simulink model "multipercursorealey"  (R2015a)
settings: Solver=ode45  StartTime=0.0  StopTime=1000.0  RelTol=1e-3
libraries: commdigbbndpm3 x2, commsink2 x2, commchan3 x1, commrandsrc2 x1
settings Model: Creator=francisco  LastModifiedBy=francisco

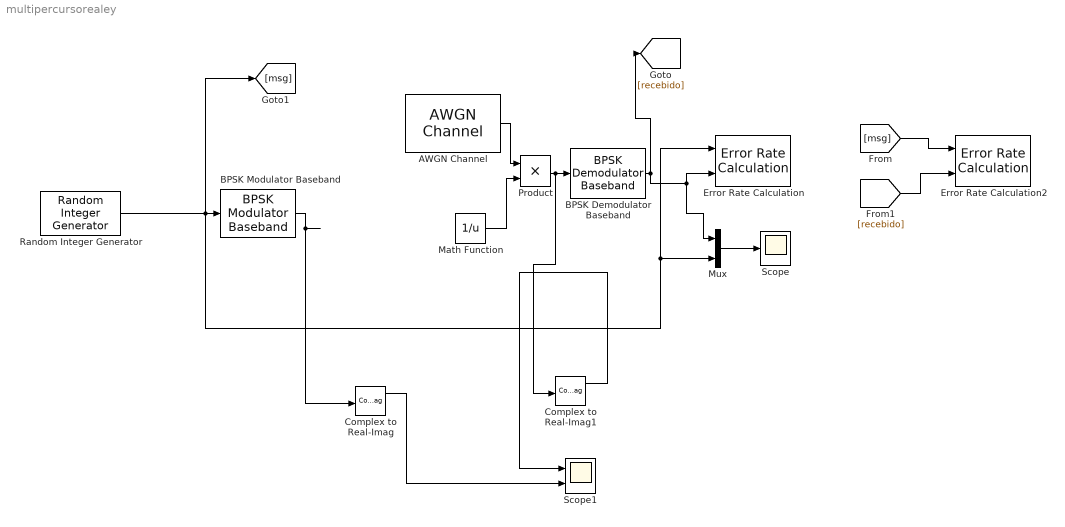
== system multipercursorealey ==
  AWGN Channel : commchan3/AWGN Channel  InputProcessing=Columns as channels (frame based)  seed=67  noiseMode="Signal to noise ratio  (Eb/No)"  EbNodB=50  EsNodB=10  SNRdB=10  bitsPerSym=1  Ps=1  Tsym=1  variance=1
  BPSK Demodulator Baseband : commdigbbndpm3/BPSK Demodulator Baseband  Ph=0  DecType=Hard decision  VarSource=Dialog  Variance=1  outDtype=Inherit via internal rule  derotateFactorWordLen=16
  BPSK Modulator Baseband : commdigbbndpm3/BPSK Modulator Baseband  Ph=0  outDtype=double  outWordLen=16  outUDDataType=sfix(16)  outFracLenMode=Best precision  outFracLen=15
  Complex to Real-Imag : ComplexToRealImag
  Complex to Real-Imag1 : ComplexToRealImag
  Error Rate Calculation : commsink2/Error Rate Calculation  N=0  st_delay=0  cp_mode=Entire frame  subframe=[]  PMode=Workspace  WsName=ErrorVec  RsMode2=off  stop=off  numErr=100  maxBits=1e6
  Error Rate Calculation2 : commsink2/Error Rate Calculation  N=0  st_delay=0  cp_mode=Entire frame  subframe=[]  PMode=Port  WsName=ErrorVec  RsMode2=off  stop=off  numErr=100  maxBits=1e6
  Math Function : Math  Operator=reciprocal  SaturateOnIntegerOverflow=on
  Mux : Mux  Inputs=2
  Product : Product
  Random Integer Generator : commrandsrc2/Random Integer Generator  mul=2  seed=37  Ts=0.01  frameBased=off  sampPerFrame=1  orient=off  outDataType=double
  Scope : Scope
      settings: Decimation=100
  Scope1 : Scope  NumInputPorts=2
      settings: YMin=-5~-5  YMax=5~5  Decimation=100
  wires:
  Random Integer Generator/1 -> [msg], BPSK Modulator Baseband/1, Error Rate Calculation/1, Mux/2
  BPSK Demodulator Baseband/1 -> Mux/1, Error Rate Calculation/2, [recebido]
  Mux/1 -> Scope/1
  BPSK Modulator Baseband/1 -> Complex to Real-Imag/1
  ? -> AWGN Channel/1
  Complex to Real-Imag1/1 -> Scope1/1
  Complex to Real-Imag/1 -> Scope1/2
  [msg] -> Error Rate Calculation2/1
  [recebido] -> Error Rate Calculation2/2
  ? -> Math Function/1
  AWGN Channel/1 -> Product/1
  Math Function/1 -> Product/2
  Product/1 -> Complex to Real-Imag1/1, BPSK Demodulator Baseband/1
